simulink library "xps_library"  (R2018a)
settings: Solver=ode45  StartTime=0.0  StopTime=10.0  RelTol=1e-3
undefined symbols (not defined in the file or in its folder): ip_name, lib_path
libraries: xbsIndex_r4 x2454, casper_library_flow_control x68, simulink x52, $bdroot x22, casper_library_misc x9
(part 3 of 27)

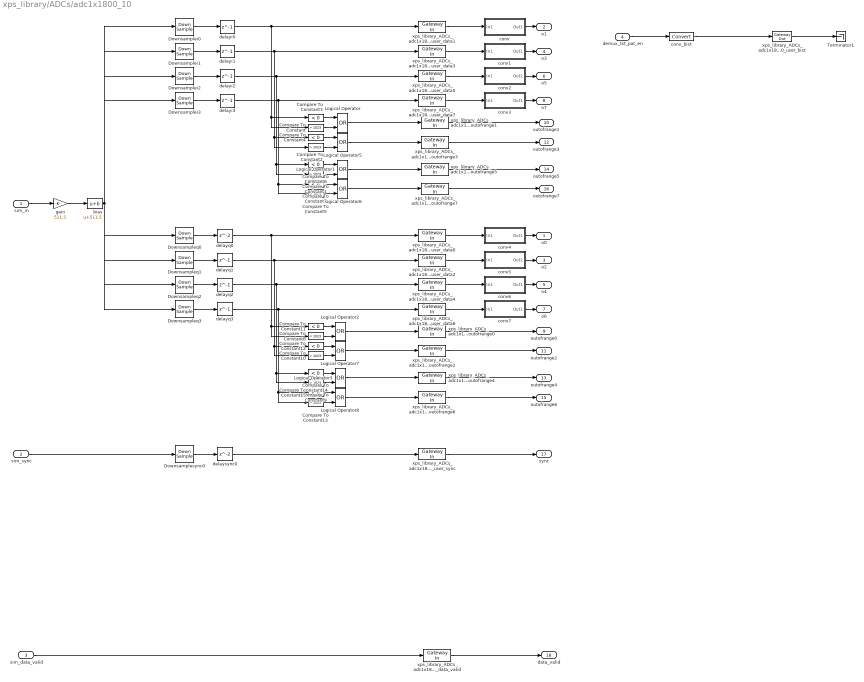
== system xps_library/ADCs/adc1x1800_10 ==
  sim_in : Inport  SampleTime=sample_period/8
  sim_sync : Inport  Port=2  SampleTime=sample_period/8
  sim_data_valid : Inport  Port=3  SampleTime=sample_period/4
  demux_tst_pat_en : Inport  Port=4  SampleTime=sample_period/8
  Compare To Constant{,1..2,5,8..10,13} (8 alike) : simulink/Logic and Bit Operations/Compare To Constant  relop=>  const=1023  OutDataTypeStr=boolean  ZeroCross=off
  Compare To Constant{3..4,6..7,11..12,14..15} (8 alike) : simulink/Logic and Bit Operations/Compare To Constant  relop=<  const=0  OutDataTypeStr=boolean  ZeroCross=off
  Downsamplei0 : DownSample  N=8  phase=1  InputProcessing=Inherited (this choice will be removed - see release notes)
  Downsamplei1 : DownSample  N=8  phase=3  InputProcessing=Inherited (this choice will be removed - see release notes)
  Downsamplei2 : DownSample  N=8  phase=5  InputProcessing=Inherited (this choice will be removed - see release notes)
  Downsamplei3 : DownSample  N=8  phase=7  InputProcessing=Inherited (this choice will be removed - see release notes)
  Downsampleq0 : DownSample  N=8  InputProcessing=Inherited (this choice will be removed - see release notes)
  Downsampleq1 : DownSample  N=8  phase=2  InputProcessing=Inherited (this choice will be removed - see release notes)
  Downsampleq2 : DownSample  N=8  phase=4  InputProcessing=Inherited (this choice will be removed - see release notes)
  Downsampleq3 : DownSample  N=8  phase=6  InputProcessing=Inherited (this choice will be removed - see release notes)
  Downsamplesync0 : DownSample  N=8  InputProcessing=Inherited (this choice will be removed - see release notes)
  Logical Operator{,1..3,5..8} (8 alike) : Logic  Operator=OR  AllPortsSameDT=off  OutDataTypeStr=boolean
  Terminator1 : Terminator
  bias : Bias  Bias=511.5  SaturateOnIntegerOverflow=on
  conv : Subsystem
  conv1 : Subsystem
  conv2 : Subsystem
  conv3 : Subsystem
  conv4 : Subsystem
  conv5 : Subsystem
  conv6 : Subsystem
  conv7 : Subsystem
  conv_bist : xbsIndex_r4/Convert  gui_display_data_type=Fixed-point  arith_type=Boolean  n_bits=8  bin_pt=0  float_type=Single  exp_bits=8  fraction_bits=24  quantization=Truncate  overflow=Wrap  en=off  latency=0  pipeline=off  dbl_ovrd=off  block_type=convert
      settings: xl_area=[0, 0, 0, 0, 0, 0, 0]
  delayi{0..3} (4 alike) : Delay  DelayLength=1  InputProcessing=Inherited
  delayq0 : Delay  InputProcessing=Inherited
  delayq1 : Delay  DelayLength=1  InputProcessing=Inherited
  delayq2 : Delay  DelayLength=1  InputProcessing=Inherited
  delayq3 : Delay  DelayLength=1  InputProcessing=Inherited
  delaysync0 : Delay  InputProcessing=Inherited
  gain : Gain  Gain=511.5  SaturateOnIntegerOverflow=on  OutDataTypeStr=Inherit: Same as input  ParamDataTypeStr=Inherit: Same as input
  xps_library_ADCs_adc1x1800_10_user_bist : xbsIndex_r4/Gateway Out  inherit_from_input=off  hdl_port=on  rows=1  columns=1  UseAsDAC=off  DACChannel='1'  interface=None  automatic_assignment=on  address_offset=hex2dec('00')  intf_name=''  intf_description=''  timing_constraint=None  locs_specified=off  LOCs={}  io_standard={}  block_type=gatewayout
      settings: infoedit="Gateway out block.  Converts Xilinx fixed point inputs into ouputs of type Simulink integer, double, or fixed point.<br><br>Hardware notes:  In hardware these blocks become top level output ports or are discarded, depending on how they are configured."  block_version=11.4
  xps_library_ADCs_adc1x1800_10_user_data{0..7} (8 alike) : xbsIndex_r4/Gateway In  gui_display_data_type=Fixed-point  arith_type=Unsigned  n_bits=10  bin_pt=0  preci_type=Single  exp_width=8  frac_width=24  rows=1  columns=1  quantization="Round  (unbiased: +/- Inf)"  overflow=Saturate  period=sample_period  UseAsADC=off  ADCChannel='1'  interface=None  automatic_assignment=on  address_offset=hex2dec('00')  intf_name=''  intf_description=''  default_value=0  timing_constraint=None  locs_specified=off  LOCs={}  io_standard={}  inherit_from_input=off  hdl_port=on  dbl_ovrd=off  block_type=gatewayin
      settings: infoedit="Gateway in block.  Converts inputs of type Simulink integer, double and fixed point to  Xilinx fixed point type.<br><br>Hardware notes:  In hardware these blocks become top level input ports."  xl_area=[0 0 0 0 8 0 0]  block_version=8.2.02
  xps_library_ADCs_adc1x1800_10_user_data_valid : xbsIndex_r4/Gateway In  gui_display_data_type=Fixed-point  arith_type=Boolean  n_bits=8  bin_pt=0  preci_type=Single  exp_width=8  frac_width=24  rows=1  columns=1  quantization="Round  (unbiased: +/- Inf)"  overflow=Saturate  period=sample_period  UseAsADC=off  ADCChannel='1'  interface=None  automatic_assignment=on  address_offset=hex2dec('00')  intf_name=''  intf_description=''  default_value=0  timing_constraint=None  locs_specified=off  LOCs={}  io_standard={}  inherit_from_input=off  hdl_port=on  dbl_ovrd=off  block_type=gatewayin
      settings: infoedit="Gateway in block.  Converts inputs of type Simulink integer, double and fixed point to  Xilinx fixed point type.<P><P>Hardware notes:  In hardware these blocks become top level input ports."  xl_area=[0 0 0 0 8 0 0]  block_version=8.2.02
  xps_library_ADCs_adc1x1800_10_user_outofrange{0..7} (8 alike) : xbsIndex_r4/Gateway In  gui_display_data_type=Fixed-point  arith_type=Boolean  n_bits=8  bin_pt=0  preci_type=Single  exp_width=8  frac_width=24  rows=1  columns=1  quantization="Round  (unbiased: +/- Inf)"  overflow=Saturate  period=sample_period  UseAsADC=off  ADCChannel='1'  interface=None  automatic_assignment=on  address_offset=hex2dec('00')  intf_name=''  intf_description=''  default_value=0  timing_constraint=None  locs_specified=off  LOCs={}  io_standard={}  inherit_from_input=off  hdl_port=on  dbl_ovrd=off  block_type=gatewayin
      settings: infoedit="Gateway in block.  Converts inputs of type Simulink integer, double and fixed point to  Xilinx fixed point type.<P><P>Hardware notes:  In hardware these blocks become top level input ports."  xl_area=[0 0 0 0 8 0 0]  block_version=8.2.02
  xps_library_ADCs_adc1x1800_10_user_sync : xbsIndex_r4/Gateway In  gui_display_data_type=Fixed-point  arith_type=Boolean  n_bits=8  bin_pt=0  preci_type=Single  exp_width=8  frac_width=24  rows=1  columns=1  quantization="Round  (unbiased: +/- Inf)"  overflow=Saturate  period=sample_period  UseAsADC=off  ADCChannel='1'  interface=None  automatic_assignment=on  address_offset=hex2dec('00')  intf_name=''  intf_description=''  default_value=0  timing_constraint=None  locs_specified=off  LOCs={}  io_standard={}  inherit_from_input=off  hdl_port=on  dbl_ovrd=off  block_type=gatewayin
      settings: infoedit="Gateway in block.  Converts inputs of type Simulink integer, double and fixed point to  Xilinx fixed point type.<P><P>Hardware notes:  In hardware these blocks become top level input ports."  xl_area=[0 0 0 0 8 0 0]  block_version=8.2.02
  o0 : Outport
  o1 : Outport  Port=2
  o2 : Outport  Port=3
  o3 : Outport  Port=4
  o4 : Outport  Port=5
  o5 : Outport  Port=6
  o6 : Outport  Port=7
  o7 : Outport  Port=8
  outofrange0 : Outport  Port=9
  outofrange1 : Outport  Port=10
  outofrange2 : Outport  Port=11
  outofrange3 : Outport  Port=12
  outofrange4 : Outport  Port=13
  outofrange5 : Outport  Port=14
  outofrange6 : Outport  Port=15
  outofrange7 : Outport  Port=16
  sync : Outport  Port=17
  data_valid : Outport  Port=18
  wires:
  delayq3/1 -> xps_library_ADCs_adc1x1800_10_user_data6/1, Compare To Constant15/1, Compare To Constant13/1
  delayq2/1 -> xps_library_ADCs_adc1x1800_10_user_data4/1, Compare To Constant14/1, Compare To Constant9/1
  delayq1/1 -> xps_library_ADCs_adc1x1800_10_user_data2/1, Compare To Constant12/1, Compare To Constant10/1
  delayi3/1 -> xps_library_ADCs_adc1x1800_10_user_data7/1, Compare To Constant7/1, Compare To Constant5/1
  delayi2/1 -> xps_library_ADCs_adc1x1800_10_user_data5/1, Compare To Constant6/1, Compare To Constant1/1
  delayi1/1 -> xps_library_ADCs_adc1x1800_10_user_data3/1, Compare To Constant2/1, Compare To Constant4/1
  Downsamplei0/1 -> delayi0/1
  xps_library_ADCs_adc1x1800_10_user_data6/1 -> conv7/1(In1)
  xps_library_ADCs_adc1x1800_10_user_data4/1 -> conv6/1(In1)
  xps_library_ADCs_adc1x1800_10_user_data2/1 -> conv5/1(In1)
  xps_library_ADCs_adc1x1800_10_user_data0/1 -> conv4/1(In1)
  xps_library_ADCs_adc1x1800_10_user_sync/1 -> sync/1
  xps_library_ADCs_adc1x1800_10_user_outofrange1/1 -> outofrange1/1
  xps_library_ADCs_adc1x1800_10_user_data7/1 -> conv3/1(In1)
  xps_library_ADCs_adc1x1800_10_user_data5/1 -> conv2/1(In1)
  xps_library_ADCs_adc1x1800_10_user_data3/1 -> conv1/1(In1)
  Downsampleq3/1 -> delayq3/1
  Downsampleq2/1 -> delayq2/1
  Downsampleq1/1 -> delayq1/1
  Downsamplei3/1 -> delayi3/1
  Downsamplei2/1 -> delayi2/1
  Downsamplei1/1 -> delayi1/1
  delayi0/1 -> xps_library_ADCs_adc1x1800_10_user_data1/1, Compare To Constant/1, Compare To Constant3/1
  Downsampleq0/1 -> delayq0/1
  delayq0/1 -> xps_library_ADCs_adc1x1800_10_user_data0/1, Compare To Constant11/1, Compare To Constant8/1
  Compare To Constant3/1 -> Logical Operator/1
  Compare To Constant/1 -> Logical Operator/2
  Compare To Constant4/1 -> Logical Operator5/1
  Compare To Constant2/1 -> Logical Operator5/2
  Logical Operator/1 -> xps_library_ADCs_adc1x1800_10_user_outofrange1/1
  Compare To Constant6/1 -> Logical Operator1/1
  Compare To Constant1/1 -> Logical Operator1/2
  Compare To Constant7/1 -> Logical Operator6/1
  Compare To Constant5/1 -> Logical Operator6/2
  Compare To Constant11/1 -> Logical Operator2/1
  Compare To Constant8/1 -> Logical Operator2/2
  Compare To Constant12/1 -> Logical Operator7/1
  Compare To Constant10/1 -> Logical Operator7/2
  Compare To Constant14/1 -> Logical Operator3/1
  Compare To Constant9/1 -> Logical Operator3/2
  Compare To Constant15/1 -> Logical Operator8/1
  Compare To Constant13/1 -> Logical Operator8/2
  sim_sync/1 -> Downsamplesync0/1
  Downsamplesync0/1 -> delaysync0/1
  delaysync0/1 -> xps_library_ADCs_adc1x1800_10_user_sync/1
  xps_library_ADCs_adc1x1800_10_user_data1/1 -> conv/1(In1)
  sim_in/1 -> gain/1
  gain/1 -> bias/1
  bias/1 -> Downsamplei0/1, Downsamplei1/1, Downsamplei2/1, Downsamplei3/1, Downsampleq0/1, Downsampleq1/1, Downsampleq2/1, Downsampleq3/1
  xps_library_ADCs_adc1x1800_10_user_outofrange3/1 -> outofrange3/1
  Logical Operator5/1 -> xps_library_ADCs_adc1x1800_10_user_outofrange3/1
  xps_library_ADCs_adc1x1800_10_user_outofrange5/1 -> outofrange5/1
  Logical Operator1/1 -> xps_library_ADCs_adc1x1800_10_user_outofrange5/1
  xps_library_ADCs_adc1x1800_10_user_outofrange7/1 -> outofrange7/1
  Logical Operator6/1 -> xps_library_ADCs_adc1x1800_10_user_outofrange7/1
  xps_library_ADCs_adc1x1800_10_user_outofrange0/1 -> outofrange0/1
  Logical Operator2/1 -> xps_library_ADCs_adc1x1800_10_user_outofrange0/1
  xps_library_ADCs_adc1x1800_10_user_outofrange2/1 -> outofrange2/1
  Logical Operator7/1 -> xps_library_ADCs_adc1x1800_10_user_outofrange2/1
  xps_library_ADCs_adc1x1800_10_user_outofrange4/1 -> outofrange4/1
  Logical Operator3/1 -> xps_library_ADCs_adc1x1800_10_user_outofrange4/1
  xps_library_ADCs_adc1x1800_10_user_outofrange6/1 -> outofrange6/1
  Logical Operator8/1 -> xps_library_ADCs_adc1x1800_10_user_outofrange6/1
  xps_library_ADCs_adc1x1800_10_user_data_valid/1 -> data_valid/1
  sim_data_valid/1 -> xps_library_ADCs_adc1x1800_10_user_data_valid/1
  demux_tst_pat_en/1 -> conv_bist/1
  xps_library_ADCs_adc1x1800_10_user_bist/1 -> Terminator1/1
  conv_bist/1 -> xps_library_ADCs_adc1x1800_10_user_bist/1
  conv/1(Out1) -> o1/1
  conv1/1(Out1) -> o3/1
  conv2/1(Out1) -> o5/1
  conv3/1(Out1) -> o7/1
  conv4/1(Out1) -> o0/1
  conv5/1(Out1) -> o2/1
  conv6/1(Out1) -> o4/1
  conv7/1(Out1) -> o6/1

== system xps_library/ADCs/adc2x14_400 ==
  conv : Subsystem
      mask help:
      | Converts an (12-bit) unsigned number to 2's complement.
      | This block should eventually be able to handle arbitrary
      | width inputs.
  conv1 : Subsystem
      mask help:
      | Converts an (12-bit) unsigned number to 2's complement.
      | This block should eventually be able to handle arbitrary
      | width inputs.
  conv2 : Subsystem
      mask help:
      | Converts an (12-bit) unsigned number to 2's complement.
      | This block should eventually be able to handle arbitrary
      | width inputs.
  conv3 : Subsystem
      mask help:
      | Converts an (12-bit) unsigned number to 2's complement.
      | This block should eventually be able to handle arbitrary
      | width inputs.
  xps_library_ADCs_adc2x14_400_user_data_i0 : xbsIndex_r4/Gateway In  gui_display_data_type=Fixed-point  arith_type=Unsigned  n_bits=14  bin_pt=0  preci_type=Single  exp_width=8  frac_width=24  rows=1  columns=1  quantization=Truncate  overflow=Wrap  period=1  UseAsADC=off  ADCChannel='1'  interface=None  automatic_assignment=on  address_offset=hex2dec('00')  intf_name=''  intf_description=''  default_value=0  timing_constraint=None  locs_specified=off  LOCs={}  io_standard={}  inherit_from_input=off  hdl_port=on  dbl_ovrd=off  block_type=gatewayin
      settings: infoedit="Gateway in block.  Converts inputs of type Simulink integer, double and fixed point to  Xilinx fixed point type.<P><P>Hardware notes:  In hardware these blocks become top level input ports."  xl_area=[0, 0, 0, 0, 0, 0, 0]  block_version=10.1.3
  xps_library_ADCs_adc2x14_400_user_data_i1 : xbsIndex_r4/Gateway In  gui_display_data_type=Fixed-point  arith_type=Unsigned  n_bits=14  bin_pt=0  preci_type=Single  exp_width=8  frac_width=24  rows=1  columns=1  quantization=Truncate  overflow=Wrap  period=1  UseAsADC=off  ADCChannel='1'  interface=None  automatic_assignment=on  address_offset=hex2dec('00')  intf_name=''  intf_description=''  default_value=0  timing_constraint=None  locs_specified=off  LOCs={}  io_standard={}  inherit_from_input=off  hdl_port=on  dbl_ovrd=off  block_type=gatewayin
      settings: infoedit="Gateway in block.  Converts inputs of type Simulink integer, double and fixed point to  Xilinx fixed point type.<P><P>Hardware notes:  In hardware these blocks become top level input ports."  xl_area=[0, 0, 0, 0, 0, 0, 0]  block_version=10.1.3
  xps_library_ADCs_adc2x14_400_user_data_q0 : xbsIndex_r4/Gateway In  gui_display_data_type=Fixed-point  arith_type=Unsigned  n_bits=14  bin_pt=0  preci_type=Single  exp_width=8  frac_width=24  rows=1  columns=1  quantization=Truncate  overflow=Wrap  period=1  UseAsADC=off  ADCChannel='1'  interface=None  automatic_assignment=on  address_offset=hex2dec('00')  intf_name=''  intf_description=''  default_value=0  timing_constraint=None  locs_specified=off  LOCs={}  io_standard={}  inherit_from_input=off  hdl_port=on  dbl_ovrd=off  block_type=gatewayin
      settings: infoedit="Gateway in block.  Converts inputs of type Simulink integer, double and fixed point to  Xilinx fixed point type.<P><P>Hardware notes:  In hardware these blocks become top level input ports."  xl_area=[0, 0, 0, 0, 0, 0, 0]  block_version=10.1.3
  xps_library_ADCs_adc2x14_400_user_data_q1 : xbsIndex_r4/Gateway In  gui_display_data_type=Fixed-point  arith_type=Unsigned  n_bits=14  bin_pt=0  preci_type=Single  exp_width=8  frac_width=24  rows=1  columns=1  quantization=Truncate  overflow=Wrap  period=1  UseAsADC=off  ADCChannel='1'  interface=None  automatic_assignment=on  address_offset=hex2dec('00')  intf_name=''  intf_description=''  default_value=0  timing_constraint=None  locs_specified=off  LOCs={}  io_standard={}  inherit_from_input=off  hdl_port=on  dbl_ovrd=off  block_type=gatewayin
      settings: infoedit="Gateway in block.  Converts inputs of type Simulink integer, double and fixed point to  Xilinx fixed point type.<P><P>Hardware notes:  In hardware these blocks become top level input ports."  xl_area=[0, 0, 0, 0, 0, 0, 0]  block_version=10.1.3
  xps_library_ADCs_adc2x14_400_user_sync : xbsIndex_r4/Gateway In  gui_display_data_type=Fixed-point  arith_type=Boolean  n_bits=1  bin_pt=0  preci_type=Single  exp_width=8  frac_width=24  rows=1  columns=1  quantization=Truncate  overflow=Wrap  period=1  UseAsADC=off  ADCChannel='1'  interface=None  automatic_assignment=on  address_offset=hex2dec('00')  intf_name=''  intf_description=''  default_value=0  timing_constraint=None  locs_specified=off  LOCs={}  io_standard={}  inherit_from_input=off  hdl_port=on  dbl_ovrd=off  block_type=gatewayin
      settings: infoedit="Gateway in block.  Converts inputs of type Simulink integer, double and fixed point to  Xilinx fixed point type.<P><P>Hardware notes:  In hardware these blocks become top level input ports."  xl_area=[0, 0, 0, 0, 0, 0, 0]  block_version=10.1.3
  data_i0 : Outport
  data_i1 : Outport  Port=2
  data_q0 : Outport  Port=3
  data_q1 : Outport  Port=4
  sync : Outport  Port=5
  wires:
  xps_library_ADCs_adc2x14_400_user_sync/1 -> sync/1
  xps_library_ADCs_adc2x14_400_user_data_i0/1 -> conv/1(In1)
  conv/1(Out1) -> data_i0/1
  xps_library_ADCs_adc2x14_400_user_data_q0/1 -> conv2/1(In1)
  conv2/1(Out1) -> data_q0/1
  xps_library_ADCs_adc2x14_400_user_data_i1/1 -> conv1/1(In1)
  conv1/1(Out1) -> data_i1/1
  xps_library_ADCs_adc2x14_400_user_data_q1/1 -> conv3/1(In1)
  conv3/1(Out1) -> data_q1/1

== system xps_library/ADCs/adc2x14_400_4x ==
  conv : Subsystem
      mask help:
      | Converts an (14-bit) unsigned number to 2's complement.
      | This block should eventually be able to handle arbitrary
      | width inputs.
  conv1 : Subsystem
      mask help:
      | Converts an (14-bit) unsigned number to 2's complement.
      | This block should eventually be able to handle arbitrary
      | width inputs.
  conv2 : Subsystem
      mask help:
      | Converts an (14-bit) unsigned number to 2's complement.
      | This block should eventually be able to handle arbitrary
      | width inputs.
  conv3 : Subsystem
      mask help:
      | Converts an (14-bit) unsigned number to 2's complement.
      | This block should eventually be able to handle arbitrary
      | width inputs.
  conv4 : Subsystem
      mask help:
      | Converts an (14-bit) unsigned number to 2's complement.
      | This block should eventually be able to handle arbitrary
      | width inputs.
  conv5 : Subsystem
      mask help:
      | Converts an (14-bit) unsigned number to 2's complement.
      | This block should eventually be able to handle arbitrary
      | width inputs.
  conv6 : Subsystem
      mask help:
      | Converts an (14-bit) unsigned number to 2's complement.
      | This block should eventually be able to handle arbitrary
      | width inputs.
  conv7 : Subsystem
      mask help:
      | Converts an (14-bit) unsigned number to 2's complement.
      | This block should eventually be able to handle arbitrary
      | width inputs.
  xps_library_ADCs_adc2x14_400_4x_user_data_i{0..3} (4 alike) : xbsIndex_r4/Gateway In  gui_display_data_type=Fixed-point  arith_type=Unsigned  n_bits=14  bin_pt=0  preci_type=Single  exp_width=8  frac_width=24  rows=1  columns=1  quantization=Truncate  overflow=Wrap  period=1  UseAsADC=off  ADCChannel='1'  interface=None  automatic_assignment=on  address_offset=hex2dec('00')  intf_name=''  intf_description=''  default_value=0  timing_constraint=None  locs_specified=off  LOCs={}  io_standard={}  inherit_from_input=off  hdl_port=on  dbl_ovrd=off  block_type=gatewayin
      settings: infoedit="Gateway in block.  Converts inputs of type Simulink integer, double and fixed point to  Xilinx fixed point type.<P><P>Hardware notes:  In hardware these blocks become top level input ports."  xl_area=[0, 0, 0, 0, 0, 0, 0]  block_version=10.1.3
  xps_library_ADCs_adc2x14_400_4x_user_data_q{0..3} (4 alike) : xbsIndex_r4/Gateway In  gui_display_data_type=Fixed-point  arith_type=Unsigned  n_bits=14  bin_pt=0  preci_type=Single  exp_width=8  frac_width=24  rows=1  columns=1  quantization=Truncate  overflow=Wrap  period=1  UseAsADC=off  ADCChannel='1'  interface=None  automatic_assignment=on  address_offset=hex2dec('00')  intf_name=''  intf_description=''  default_value=0  timing_constraint=None  locs_specified=off  LOCs={}  io_standard={}  inherit_from_input=off  hdl_port=on  dbl_ovrd=off  block_type=gatewayin
      settings: infoedit="Gateway in block.  Converts inputs of type Simulink integer, double and fixed point to  Xilinx fixed point type.<P><P>Hardware notes:  In hardware these blocks become top level input ports."  xl_area=[0, 0, 0, 0, 0, 0, 0]  block_version=10.1.3
  xps_library_ADCs_adc2x14_400_4x_user_sync : xbsIndex_r4/Gateway In  gui_display_data_type=Fixed-point  arith_type=Boolean  n_bits=1  bin_pt=0  preci_type=Single  exp_width=8  frac_width=24  rows=1  columns=1  quantization=Truncate  overflow=Wrap  period=1  UseAsADC=off  ADCChannel='1'  interface=None  automatic_assignment=on  address_offset=hex2dec('00')  intf_name=''  intf_description=''  default_value=0  timing_constraint=None  locs_specified=off  LOCs={}  io_standard={}  inherit_from_input=off  hdl_port=on  dbl_ovrd=off  block_type=gatewayin
      settings: infoedit="Gateway in block.  Converts inputs of type Simulink integer, double and fixed point to  Xilinx fixed point type.<P><P>Hardware notes:  In hardware these blocks become top level input ports."  xl_area=[0, 0, 0, 0, 0, 0, 0]  block_version=10.1.3
  data_i0 : Outport
  data_i1 : Outport  Port=2
  data_i2 : Outport  Port=3
  data_i3 : Outport  Port=4
  data_q0 : Outport  Port=5
  data_q1 : Outport  Port=6
  data_q2 : Outport  Port=7
  data_q3 : Outport  Port=8
  sync : Outport  Port=9
  wires:
  conv5/1(Out1) -> data_q1/1
  xps_library_ADCs_adc2x14_400_4x_user_data_q1/1 -> conv5/1(In1)
  conv1/1(Out1) -> data_i1/1
  xps_library_ADCs_adc2x14_400_4x_user_data_i1/1 -> conv1/1(In1)
  conv4/1(Out1) -> data_q0/1
  xps_library_ADCs_adc2x14_400_4x_user_data_q0/1 -> conv4/1(In1)
  conv/1(Out1) -> data_i0/1
  xps_library_ADCs_adc2x14_400_4x_user_data_i0/1 -> conv/1(In1)
  xps_library_ADCs_adc2x14_400_4x_user_sync/1 -> sync/1
  conv2/1(Out1) -> data_i2/1
  xps_library_ADCs_adc2x14_400_4x_user_data_i2/1 -> conv2/1(In1)
  conv3/1(Out1) -> data_i3/1
  xps_library_ADCs_adc2x14_400_4x_user_data_i3/1 -> conv3/1(In1)
  conv6/1(Out1) -> data_q2/1
  xps_library_ADCs_adc2x14_400_4x_user_data_q2/1 -> conv6/1(In1)
  conv7/1(Out1) -> data_q3/1
  xps_library_ADCs_adc2x14_400_4x_user_data_q3/1 -> conv7/1(In1)

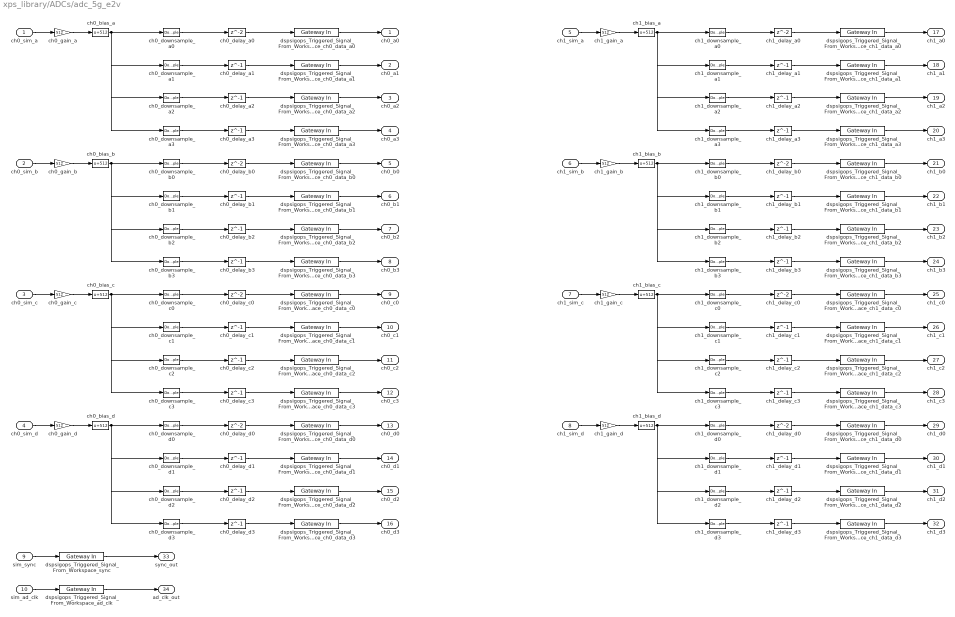
== system xps_library/ADCs/adc_5g_e2v ==
  ch0_sim_a : Inport
  ch0_sim_b : Inport  Port=2
  ch0_sim_c : Inport  Port=3
  ch0_sim_d : Inport  Port=4
  ch1_sim_a : Inport  Port=5
  ch1_sim_b : Inport  Port=6
  ch1_sim_c : Inport  Port=7
  ch1_sim_d : Inport  Port=8
  sim_sync : Inport  Port=9
  sim_ad_clk : Inport  Port=10
  ch0_bias_a : Bias  Bias=512  SaturateOnIntegerOverflow=on
  ch0_bias_b : Bias  Bias=512  SaturateOnIntegerOverflow=on
  ch0_bias_c : Bias  Bias=512  SaturateOnIntegerOverflow=on
  ch0_bias_d : Bias  Bias=512  SaturateOnIntegerOverflow=on
  ch0_delay_a0 : Delay  InitialCondition=0  InputProcessing=Inherited
  ch0_delay_a1 : Delay  DelayLength=1  InitialCondition=0  InputProcessing=Inherited
  ch0_delay_a2 : Delay  DelayLength=1  InitialCondition=0  InputProcessing=Inherited
  ch0_delay_a3 : Delay  DelayLength=1  InitialCondition=0  InputProcessing=Inherited
  ch0_delay_b0 : Delay  InitialCondition=0  InputProcessing=Inherited
  ch0_delay_b1 : Delay  DelayLength=1  InitialCondition=0  InputProcessing=Inherited
  ch0_delay_b2 : Delay  DelayLength=1  InitialCondition=0  InputProcessing=Inherited
  ch0_delay_b3 : Delay  DelayLength=1  InitialCondition=0  InputProcessing=Inherited
  ch0_delay_c0 : Delay  InitialCondition=0  InputProcessing=Inherited
  ch0_delay_c1 : Delay  DelayLength=1  InitialCondition=0  InputProcessing=Inherited
  ch0_delay_c2 : Delay  DelayLength=1  InitialCondition=0  InputProcessing=Inherited
  ch0_delay_c3 : Delay  DelayLength=1  InitialCondition=0  InputProcessing=Inherited
  ch0_delay_d0 : Delay  InitialCondition=0  InputProcessing=Inherited
  ch0_delay_d1 : Delay  DelayLength=1  InitialCondition=0  InputProcessing=Inherited
  ch0_delay_d2 : Delay  DelayLength=1  InitialCondition=0  InputProcessing=Inherited
  ch0_delay_d3 : Delay  DelayLength=1  InitialCondition=0  InputProcessing=Inherited
  ch0_downsample_a0 : DownSample  N=4  RateOptions=Allow multirate processing
  ch0_downsample_a1 : DownSample  N=4  phase=1  RateOptions=Allow multirate processing
  ch0_downsample_a2 : DownSample  N=4  phase=2  RateOptions=Allow multirate processing
  ch0_downsample_a3 : DownSample  N=4  phase=3  RateOptions=Allow multirate processing
  ch0_downsample_b0 : DownSample  N=4  RateOptions=Allow multirate processing
  ch0_downsample_b1 : DownSample  N=4  phase=1  RateOptions=Allow multirate processing
  ch0_downsample_b2 : DownSample  N=4  phase=2  RateOptions=Allow multirate processing
  ch0_downsample_b3 : DownSample  N=4  phase=3  RateOptions=Allow multirate processing
  ch0_downsample_c0 : DownSample  N=4  RateOptions=Allow multirate processing
  ch0_downsample_c1 : DownSample  N=4  phase=1  RateOptions=Allow multirate processing
  ch0_downsample_c2 : DownSample  N=4  phase=2  RateOptions=Allow multirate processing
  ch0_downsample_c3 : DownSample  N=4  phase=3  RateOptions=Allow multirate processing
  ch0_downsample_d0 : DownSample  N=4  RateOptions=Allow multirate processing
  ch0_downsample_d1 : DownSample  N=4  phase=1  RateOptions=Allow multirate processing
  ch0_downsample_d2 : DownSample  N=4  phase=2  RateOptions=Allow multirate processing
  ch0_downsample_d3 : DownSample  N=4  phase=3  RateOptions=Allow multirate processing
  ch0_gain_a : Gain  Gain=512  SaturateOnIntegerOverflow=on  OutDataTypeStr=Inherit: Same as input  ParamDataTypeStr=Inherit: Same as input
  ch0_gain_b : Gain  Gain=512  SaturateOnIntegerOverflow=on  OutDataTypeStr=Inherit: Same as input  ParamDataTypeStr=Inherit: Same as input
  ch0_gain_c : Gain  Gain=512  SaturateOnIntegerOverflow=on  OutDataTypeStr=Inherit: Same as input  ParamDataTypeStr=Inherit: Same as input
  ch0_gain_d : Gain  Gain=512  SaturateOnIntegerOverflow=on  OutDataTypeStr=Inherit: Same as input  ParamDataTypeStr=Inherit: Same as input
  ch1_bias_a : Bias  Bias=512  SaturateOnIntegerOverflow=on
  ch1_bias_b : Bias  Bias=512  SaturateOnIntegerOverflow=on
  ch1_bias_c : Bias  Bias=512  SaturateOnIntegerOverflow=on
  ch1_bias_d : Bias  Bias=512  SaturateOnIntegerOverflow=on
  ch1_delay_a0 : Delay  InitialCondition=0  InputProcessing=Inherited
  ch1_delay_a1 : Delay  DelayLength=1  InitialCondition=0  InputProcessing=Inherited
  ch1_delay_a2 : Delay  DelayLength=1  InitialCondition=0  InputProcessing=Inherited
  ch1_delay_a3 : Delay  DelayLength=1  InitialCondition=0  InputProcessing=Inherited
  ch1_delay_b0 : Delay  InitialCondition=0  InputProcessing=Inherited
  ch1_delay_b1 : Delay  DelayLength=1  InitialCondition=0  InputProcessing=Inherited
  ch1_delay_b2 : Delay  DelayLength=1  InitialCondition=0  InputProcessing=Inherited
  ch1_delay_b3 : Delay  DelayLength=1  InitialCondition=0  InputProcessing=Inherited
  ch1_delay_c0 : Delay  InitialCondition=0  InputProcessing=Inherited
  ch1_delay_c1 : Delay  DelayLength=1  InitialCondition=0  InputProcessing=Inherited
  ch1_delay_c2 : Delay  DelayLength=1  InitialCondition=0  InputProcessing=Inherited
  ch1_delay_c3 : Delay  DelayLength=1  InitialCondition=0  InputProcessing=Inherited
  ch1_delay_d0 : Delay  InitialCondition=0  InputProcessing=Inherited
  ch1_delay_d1 : Delay  DelayLength=1  InitialCondition=0  InputProcessing=Inherited
  ch1_delay_d2 : Delay  DelayLength=1  InitialCondition=0  InputProcessing=Inherited
  ch1_delay_d3 : Delay  DelayLength=1  InitialCondition=0  InputProcessing=Inherited
  ch1_downsample_a0 : DownSample  N=4  RateOptions=Allow multirate processing
  ch1_downsample_a1 : DownSample  N=4  phase=1  RateOptions=Allow multirate processing
  ch1_downsample_a2 : DownSample  N=4  phase=2  RateOptions=Allow multirate processing
  ch1_downsample_a3 : DownSample  N=4  phase=3  RateOptions=Allow multirate processing
  ch1_downsample_b0 : DownSample  N=4  RateOptions=Allow multirate processing
  ch1_downsample_b1 : DownSample  N=4  phase=1  RateOptions=Allow multirate processing
  ch1_downsample_b2 : DownSample  N=4  phase=2  RateOptions=Allow multirate processing
  ch1_downsample_b3 : DownSample  N=4  phase=3  RateOptions=Allow multirate processing
  ch1_downsample_c0 : DownSample  N=4  RateOptions=Allow multirate processing
  ch1_downsample_c1 : DownSample  N=4  phase=1  RateOptions=Allow multirate processing
  ch1_downsample_c2 : DownSample  N=4  phase=2  RateOptions=Allow multirate processing
  ch1_downsample_c3 : DownSample  N=4  phase=3  RateOptions=Allow multirate processing
  ch1_downsample_d0 : DownSample  N=4  RateOptions=Allow multirate processing
  ch1_downsample_d1 : DownSample  N=4  phase=1  RateOptions=Allow multirate processing
  ch1_downsample_d2 : DownSample  N=4  phase=2  RateOptions=Allow multirate processing
  ch1_downsample_d3 : DownSample  N=4  phase=3  RateOptions=Allow multirate processing
  ch1_gain_a : Gain  Gain=512  SaturateOnIntegerOverflow=on  OutDataTypeStr=Inherit: Same as input  ParamDataTypeStr=Inherit: Same as input
  ch1_gain_b : Gain  Gain=512  SaturateOnIntegerOverflow=on  OutDataTypeStr=Inherit: Same as input  ParamDataTypeStr=Inherit: Same as input
  ch1_gain_c : Gain  Gain=512  SaturateOnIntegerOverflow=on  OutDataTypeStr=Inherit: Same as input  ParamDataTypeStr=Inherit: Same as input
  ch1_gain_d : Gain  Gain=512  SaturateOnIntegerOverflow=on  OutDataTypeStr=Inherit: Same as input  ParamDataTypeStr=Inherit: Same as input
  dspsigops_Triggered_Signal_From_Workspace_ad_clk : xbsIndex_r4/Gateway In  gui_display_data_type=Fixed-point  arith_type=Boolean  n_bits=16  bin_pt=14  preci_type=Single  exp_width=8  frac_width=24  rows=1  columns=1  quantization="Round  (unbiased: +/- Inf)"  overflow=Saturate  period=1  UseAsADC=off  ADCChannel='1'  interface=None  automatic_assignment=on  address_offset=hex2dec('00')  intf_name=''  intf_description=''  default_value=0  timing_constraint=None  locs_specified=off  LOCs={}  io_standard={}  inherit_from_input=off  hdl_port=on  dbl_ovrd=off  block_type=gatewayin
  dspsigops_Triggered_Signal_From_Workspace_ch0_data_a{0..3} (4 alike) : xbsIndex_r4/Gateway In  gui_display_data_type=Fixed-point  arith_type=Unsigned  n_bits=10  bin_pt=0  preci_type=Single  exp_width=8  frac_width=24  rows=1  columns=1  quantization=Truncate  overflow=Wrap  period=1  UseAsADC=off  ADCChannel='1'  interface=None  automatic_assignment=on  address_offset=hex2dec('00')  intf_name=''  intf_description=''  default_value=0  timing_constraint=None  locs_specified=off  LOCs={}  io_standard={}  inherit_from_input=off  hdl_port=on  dbl_ovrd=off  block_type=gatewayin
  dspsigops_Triggered_Signal_From_Workspace_ch0_data_b{0..3} (4 alike) : xbsIndex_r4/Gateway In  gui_display_data_type=Fixed-point  arith_type=Unsigned  n_bits=10  bin_pt=0  preci_type=Single  exp_width=8  frac_width=24  rows=1  columns=1  quantization=Truncate  overflow=Wrap  period=1  UseAsADC=off  ADCChannel='1'  interface=None  automatic_assignment=on  address_offset=hex2dec('00')  intf_name=''  intf_description=''  default_value=0  timing_constraint=None  locs_specified=off  LOCs={}  io_standard={}  inherit_from_input=off  hdl_port=on  dbl_ovrd=off  block_type=gatewayin
  dspsigops_Triggered_Signal_From_Workspace_ch0_data_c{0..3} (4 alike) : xbsIndex_r4/Gateway In  gui_display_data_type=Fixed-point  arith_type=Unsigned  n_bits=10  bin_pt=0  preci_type=Single  exp_width=8  frac_width=24  rows=1  columns=1  quantization=Truncate  overflow=Wrap  period=1  UseAsADC=off  ADCChannel='1'  interface=None  automatic_assignment=on  address_offset=hex2dec('00')  intf_name=''  intf_description=''  default_value=0  timing_constraint=None  locs_specified=off  LOCs={}  io_standard={}  inherit_from_input=off  hdl_port=on  dbl_ovrd=off  block_type=gatewayin
  dspsigops_Triggered_Signal_From_Workspace_ch0_data_d{0..3} (4 alike) : xbsIndex_r4/Gateway In  gui_display_data_type=Fixed-point  arith_type=Unsigned  n_bits=10  bin_pt=0  preci_type=Single  exp_width=8  frac_width=24  rows=1  columns=1  quantization=Truncate  overflow=Wrap  period=1  UseAsADC=off  ADCChannel='1'  interface=None  automatic_assignment=on  address_offset=hex2dec('00')  intf_name=''  intf_description=''  default_value=0  timing_constraint=None  locs_specified=off  LOCs={}  io_standard={}  inherit_from_input=off  hdl_port=on  dbl_ovrd=off  block_type=gatewayin
  dspsigops_Triggered_Signal_From_Workspace_ch1_data_a{0..3} (4 alike) : xbsIndex_r4/Gateway In  gui_display_data_type=Fixed-point  arith_type=Unsigned  n_bits=10  bin_pt=0  preci_type=Single  exp_width=8  frac_width=24  rows=1  columns=1  quantization=Truncate  overflow=Wrap  period=1  UseAsADC=off  ADCChannel='1'  interface=None  automatic_assignment=on  address_offset=hex2dec('00')  intf_name=''  intf_description=''  default_value=0  timing_constraint=None  locs_specified=off  LOCs={}  io_standard={}  inherit_from_input=off  hdl_port=on  dbl_ovrd=off  block_type=gatewayin
  dspsigops_Triggered_Signal_From_Workspace_ch1_data_b{0..3} (4 alike) : xbsIndex_r4/Gateway In  gui_display_data_type=Fixed-point  arith_type=Unsigned  n_bits=10  bin_pt=0  preci_type=Single  exp_width=8  frac_width=24  rows=1  columns=1  quantization=Truncate  overflow=Wrap  period=1  UseAsADC=off  ADCChannel='1'  interface=None  automatic_assignment=on  address_offset=hex2dec('00')  intf_name=''  intf_description=''  default_value=0  timing_constraint=None  locs_specified=off  LOCs={}  io_standard={}  inherit_from_input=off  hdl_port=on  dbl_ovrd=off  block_type=gatewayin
  dspsigops_Triggered_Signal_From_Workspace_ch1_data_c{0..3} (4 alike) : xbsIndex_r4/Gateway In  gui_display_data_type=Fixed-point  arith_type=Unsigned  n_bits=10  bin_pt=0  preci_type=Single  exp_width=8  frac_width=24  rows=1  columns=1  quantization=Truncate  overflow=Wrap  period=1  UseAsADC=off  ADCChannel='1'  interface=None  automatic_assignment=on  address_offset=hex2dec('00')  intf_name=''  intf_description=''  default_value=0  timing_constraint=None  locs_specified=off  LOCs={}  io_standard={}  inherit_from_input=off  hdl_port=on  dbl_ovrd=off  block_type=gatewayin
  dspsigops_Triggered_Signal_From_Workspace_ch1_data_d{0..3} (4 alike) : xbsIndex_r4/Gateway In  gui_display_data_type=Fixed-point  arith_type=Unsigned  n_bits=10  bin_pt=0  preci_type=Single  exp_width=8  frac_width=24  rows=1  columns=1  quantization=Truncate  overflow=Wrap  period=1  UseAsADC=off  ADCChannel='1'  interface=None  automatic_assignment=on  address_offset=hex2dec('00')  intf_name=''  intf_description=''  default_value=0  timing_constraint=None  locs_specified=off  LOCs={}  io_standard={}  inherit_from_input=off  hdl_port=on  dbl_ovrd=off  block_type=gatewayin
  dspsigops_Triggered_Signal_From_Workspace_sync : xbsIndex_r4/Gateway In  gui_display_data_type=Fixed-point  arith_type=Boolean  n_bits=16  bin_pt=14  preci_type=Single  exp_width=8  frac_width=24  rows=1  columns=1  quantization="Round  (unbiased: +/- Inf)"  overflow=Saturate  period=1  UseAsADC=off  ADCChannel='1'  interface=None  automatic_assignment=on  address_offset=hex2dec('00')  intf_name=''  intf_description=''  default_value=0  timing_constraint=None  locs_specified=off  LOCs={}  io_standard={}  inherit_from_input=off  hdl_port=on  dbl_ovrd=off  block_type=gatewayin
  ch0_a0 : Outport
  ch0_a1 : Outport  Port=2
  ch0_a2 : Outport  Port=3
  ch0_a3 : Outport  Port=4
  ch0_b0 : Outport  Port=5
  ch0_b1 : Outport  Port=6
  ch0_b2 : Outport  Port=7
  ch0_b3 : Outport  Port=8
  ch0_c0 : Outport  Port=9
  ch0_c1 : Outport  Port=10
  ch0_c2 : Outport  Port=11
  ch0_c3 : Outport  Port=12
  ch0_d0 : Outport  Port=13
  ch0_d1 : Outport  Port=14
  ch0_d2 : Outport  Port=15
  ch0_d3 : Outport  Port=16
  ch1_a0 : Outport  Port=17
  ch1_a1 : Outport  Port=18
  ch1_a2 : Outport  Port=19
  ch1_a3 : Outport  Port=20
  ch1_b0 : Outport  Port=21
  ch1_b1 : Outport  Port=22
  ch1_b2 : Outport  Port=23
  ch1_b3 : Outport  Port=24
  ch1_c0 : Outport  Port=25
  ch1_c1 : Outport  Port=26
  ch1_c2 : Outport  Port=27
  ch1_c3 : Outport  Port=28
  ch1_d0 : Outport  Port=29
  ch1_d1 : Outport  Port=30
  ch1_d2 : Outport  Port=31
  ch1_d3 : Outport  Port=32
  sync_out : Outport  Port=33
  ad_clk_out : Outport  Port=34
  wires:
  ch0_sim_a/1 -> ch0_gain_a/1
  ch0_gain_a/1 -> ch0_bias_a/1
  ch0_bias_a/1 -> ch0_downsample_a0/1, ch0_downsample_a1/1, ch0_downsample_a2/1, ch0_downsample_a3/1
  ch0_downsample_a0/1 -> ch0_delay_a0/1
  ch0_delay_a0/1 -> dspsigops_Triggered_Signal_From_Workspace_ch0_data_a0/1
  dspsigops_Triggered_Signal_From_Workspace_ch0_data_a0/1 -> ch0_a0/1
  ch0_downsample_a1/1 -> ch0_delay_a1/1
  ch0_delay_a1/1 -> dspsigops_Triggered_Signal_From_Workspace_ch0_data_a1/1
  dspsigops_Triggered_Signal_From_Workspace_ch0_data_a1/1 -> ch0_a1/1
  ch0_downsample_a2/1 -> ch0_delay_a2/1
  ch0_delay_a2/1 -> dspsigops_Triggered_Signal_From_Workspace_ch0_data_a2/1
  dspsigops_Triggered_Signal_From_Workspace_ch0_data_a2/1 -> ch0_a2/1
  ch0_downsample_a3/1 -> ch0_delay_a3/1
  ch0_delay_a3/1 -> dspsigops_Triggered_Signal_From_Workspace_ch0_data_a3/1
  dspsigops_Triggered_Signal_From_Workspace_ch0_data_a3/1 -> ch0_a3/1
  ch0_sim_b/1 -> ch0_gain_b/1
  ch0_gain_b/1 -> ch0_bias_b/1
  ch0_bias_b/1 -> ch0_downsample_b0/1, ch0_downsample_b1/1, ch0_downsample_b2/1, ch0_downsample_b3/1
  ch0_downsample_b0/1 -> ch0_delay_b0/1
  ch0_delay_b0/1 -> dspsigops_Triggered_Signal_From_Workspace_ch0_data_b0/1
  dspsigops_Triggered_Signal_From_Workspace_ch0_data_b0/1 -> ch0_b0/1
  ch0_downsample_b1/1 -> ch0_delay_b1/1
  ch0_delay_b1/1 -> dspsigops_Triggered_Signal_From_Workspace_ch0_data_b1/1
  dspsigops_Triggered_Signal_From_Workspace_ch0_data_b1/1 -> ch0_b1/1
  ch0_downsample_b2/1 -> ch0_delay_b2/1
  ch0_delay_b2/1 -> dspsigops_Triggered_Signal_From_Workspace_ch0_data_b2/1
  dspsigops_Triggered_Signal_From_Workspace_ch0_data_b2/1 -> ch0_b2/1
  ch0_downsample_b3/1 -> ch0_delay_b3/1
  ch0_delay_b3/1 -> dspsigops_Triggered_Signal_From_Workspace_ch0_data_b3/1
  dspsigops_Triggered_Signal_From_Workspace_ch0_data_b3/1 -> ch0_b3/1
  ch0_sim_c/1 -> ch0_gain_c/1
  ch0_gain_c/1 -> ch0_bias_c/1
  ch0_bias_c/1 -> ch0_downsample_c0/1, ch0_downsample_c1/1, ch0_downsample_c2/1, ch0_downsample_c3/1
  ch0_downsample_c0/1 -> ch0_delay_c0/1
  ch0_delay_c0/1 -> dspsigops_Triggered_Signal_From_Workspace_ch0_data_c0/1
  dspsigops_Triggered_Signal_From_Workspace_ch0_data_c0/1 -> ch0_c0/1
  ch0_downsample_c1/1 -> ch0_delay_c1/1
  ch0_delay_c1/1 -> dspsigops_Triggered_Signal_From_Workspace_ch0_data_c1/1
  dspsigops_Triggered_Signal_From_Workspace_ch0_data_c1/1 -> ch0_c1/1
  ch0_downsample_c2/1 -> ch0_delay_c2/1
  ch0_delay_c2/1 -> dspsigops_Triggered_Signal_From_Workspace_ch0_data_c2/1
  dspsigops_Triggered_Signal_From_Workspace_ch0_data_c2/1 -> ch0_c2/1
  ch0_downsample_c3/1 -> ch0_delay_c3/1
  ch0_delay_c3/1 -> dspsigops_Triggered_Signal_From_Workspace_ch0_data_c3/1
  dspsigops_Triggered_Signal_From_Workspace_ch0_data_c3/1 -> ch0_c3/1
  ch0_sim_d/1 -> ch0_gain_d/1
  ch0_gain_d/1 -> ch0_bias_d/1
  ch0_bias_d/1 -> ch0_downsample_d0/1, ch0_downsample_d1/1, ch0_downsample_d2/1, ch0_downsample_d3/1
  ch0_downsample_d0/1 -> ch0_delay_d0/1
  ch0_delay_d0/1 -> dspsigops_Triggered_Signal_From_Workspace_ch0_data_d0/1
  dspsigops_Triggered_Signal_From_Workspace_ch0_data_d0/1 -> ch0_d0/1
  ch0_downsample_d1/1 -> ch0_delay_d1/1
  ch0_delay_d1/1 -> dspsigops_Triggered_Signal_From_Workspace_ch0_data_d1/1
  dspsigops_Triggered_Signal_From_Workspace_ch0_data_d1/1 -> ch0_d1/1
  ch0_downsample_d2/1 -> ch0_delay_d2/1
  ch0_delay_d2/1 -> dspsigops_Triggered_Signal_From_Workspace_ch0_data_d2/1
  dspsigops_Triggered_Signal_From_Workspace_ch0_data_d2/1 -> ch0_d2/1
  ch0_downsample_d3/1 -> ch0_delay_d3/1
  ch0_delay_d3/1 -> dspsigops_Triggered_Signal_From_Workspace_ch0_data_d3/1
  dspsigops_Triggered_Signal_From_Workspace_ch0_data_d3/1 -> ch0_d3/1
  ch1_sim_a/1 -> ch1_gain_a/1
  ch1_gain_a/1 -> ch1_bias_a/1
  ch1_bias_a/1 -> ch1_downsample_a0/1, ch1_downsample_a1/1, ch1_downsample_a2/1, ch1_downsample_a3/1
  ch1_downsample_a0/1 -> ch1_delay_a0/1
  ch1_delay_a0/1 -> dspsigops_Triggered_Signal_From_Workspace_ch1_data_a0/1
  dspsigops_Triggered_Signal_From_Workspace_ch1_data_a0/1 -> ch1_a0/1
  ch1_downsample_a1/1 -> ch1_delay_a1/1
  ch1_delay_a1/1 -> dspsigops_Triggered_Signal_From_Workspace_ch1_data_a1/1
  dspsigops_Triggered_Signal_From_Workspace_ch1_data_a1/1 -> ch1_a1/1
  ch1_downsample_a2/1 -> ch1_delay_a2/1
  ch1_delay_a2/1 -> dspsigops_Triggered_Signal_From_Workspace_ch1_data_a2/1
  dspsigops_Triggered_Signal_From_Workspace_ch1_data_a2/1 -> ch1_a2/1
  ch1_downsample_a3/1 -> ch1_delay_a3/1
  ch1_delay_a3/1 -> dspsigops_Triggered_Signal_From_Workspace_ch1_data_a3/1
  dspsigops_Triggered_Signal_From_Workspace_ch1_data_a3/1 -> ch1_a3/1
  ch1_sim_b/1 -> ch1_gain_b/1
  ch1_gain_b/1 -> ch1_bias_b/1
  ch1_bias_b/1 -> ch1_downsample_b0/1, ch1_downsample_b1/1, ch1_downsample_b2/1, ch1_downsample_b3/1
  ch1_downsample_b0/1 -> ch1_delay_b0/1
  ch1_delay_b0/1 -> dspsigops_Triggered_Signal_From_Workspace_ch1_data_b0/1
  dspsigops_Triggered_Signal_From_Workspace_ch1_data_b0/1 -> ch1_b0/1
  ch1_downsample_b1/1 -> ch1_delay_b1/1
  ch1_delay_b1/1 -> dspsigops_Triggered_Signal_From_Workspace_ch1_data_b1/1
  dspsigops_Triggered_Signal_From_Workspace_ch1_data_b1/1 -> ch1_b1/1
  ch1_downsample_b2/1 -> ch1_delay_b2/1
  ch1_delay_b2/1 -> dspsigops_Triggered_Signal_From_Workspace_ch1_data_b2/1
  dspsigops_Triggered_Signal_From_Workspace_ch1_data_b2/1 -> ch1_b2/1
  ch1_downsample_b3/1 -> ch1_delay_b3/1
  ch1_delay_b3/1 -> dspsigops_Triggered_Signal_From_Workspace_ch1_data_b3/1
  dspsigops_Triggered_Signal_From_Workspace_ch1_data_b3/1 -> ch1_b3/1
  ch1_sim_c/1 -> ch1_gain_c/1
  ch1_gain_c/1 -> ch1_bias_c/1
  ch1_bias_c/1 -> ch1_downsample_c0/1, ch1_downsample_c1/1, ch1_downsample_c2/1, ch1_downsample_c3/1
  ch1_downsample_c0/1 -> ch1_delay_c0/1
  ch1_delay_c0/1 -> dspsigops_Triggered_Signal_From_Workspace_ch1_data_c0/1
  dspsigops_Triggered_Signal_From_Workspace_ch1_data_c0/1 -> ch1_c0/1
  ch1_downsample_c1/1 -> ch1_delay_c1/1
  ch1_delay_c1/1 -> dspsigops_Triggered_Signal_From_Workspace_ch1_data_c1/1
  dspsigops_Triggered_Signal_From_Workspace_ch1_data_c1/1 -> ch1_c1/1
  ch1_downsample_c2/1 -> ch1_delay_c2/1
  ch1_delay_c2/1 -> dspsigops_Triggered_Signal_From_Workspace_ch1_data_c2/1
  dspsigops_Triggered_Signal_From_Workspace_ch1_data_c2/1 -> ch1_c2/1
  ch1_downsample_c3/1 -> ch1_delay_c3/1
  ch1_delay_c3/1 -> dspsigops_Triggered_Signal_From_Workspace_ch1_data_c3/1
  dspsigops_Triggered_Signal_From_Workspace_ch1_data_c3/1 -> ch1_c3/1
  ch1_sim_d/1 -> ch1_gain_d/1
  ch1_gain_d/1 -> ch1_bias_d/1
  ch1_bias_d/1 -> ch1_downsample_d0/1, ch1_downsample_d1/1, ch1_downsample_d2/1, ch1_downsample_d3/1
  ch1_downsample_d0/1 -> ch1_delay_d0/1
  ch1_delay_d0/1 -> dspsigops_Triggered_Signal_From_Workspace_ch1_data_d0/1
  dspsigops_Triggered_Signal_From_Workspace_ch1_data_d0/1 -> ch1_d0/1
  ch1_downsample_d1/1 -> ch1_delay_d1/1
  ch1_delay_d1/1 -> dspsigops_Triggered_Signal_From_Workspace_ch1_data_d1/1
  dspsigops_Triggered_Signal_From_Workspace_ch1_data_d1/1 -> ch1_d1/1
  ch1_downsample_d2/1 -> ch1_delay_d2/1
  ch1_delay_d2/1 -> dspsigops_Triggered_Signal_From_Workspace_ch1_data_d2/1
  dspsigops_Triggered_Signal_From_Workspace_ch1_data_d2/1 -> ch1_d2/1
  ch1_downsample_d3/1 -> ch1_delay_d3/1
  ch1_delay_d3/1 -> dspsigops_Triggered_Signal_From_Workspace_ch1_data_d3/1
  dspsigops_Triggered_Signal_From_Workspace_ch1_data_d3/1 -> ch1_d3/1
  sim_sync/1 -> dspsigops_Triggered_Signal_From_Workspace_sync/1
  dspsigops_Triggered_Signal_From_Workspace_sync/1 -> sync_out/1
  sim_ad_clk/1 -> dspsigops_Triggered_Signal_From_Workspace_ad_clk/1
  dspsigops_Triggered_Signal_From_Workspace_ad_clk/1 -> ad_clk_out/1

== system xps_library/ADCs/adc_mkid ==
  conv : Subsystem
      mask help:
      | Converts an (12-bit) unsigned number to 2's complement.
      | This block should eventually be able to handle arbitrary
      | width inputs.
  conv1 : Subsystem
      mask help:
      | Converts an (12-bit) unsigned number to 2's complement.
      | This block should eventually be able to handle arbitrary
      | width inputs.
  conv2 : Subsystem
      mask help:
      | Converts an (12-bit) unsigned number to 2's complement.
      | This block should eventually be able to handle arbitrary
      | width inputs.
  conv3 : Subsystem
      mask help:
      | Converts an (12-bit) unsigned number to 2's complement.
      | This block should eventually be able to handle arbitrary
      | width inputs.
  xps_library_ADCs_adc_mkid_user_data_i0 : xbsIndex_r4/Gateway In  gui_display_data_type=Fixed-point  arith_type=Unsigned  n_bits=12  bin_pt=0  preci_type=Single  exp_width=8  frac_width=24  rows=1  columns=1  quantization=Truncate  overflow=Wrap  period=1  UseAsADC=off  ADCChannel='1'  interface=None  automatic_assignment=on  address_offset=hex2dec('00')  intf_name=''  intf_description=''  default_value=0  timing_constraint=None  locs_specified=off  LOCs={}  io_standard={}  inherit_from_input=off  hdl_port=on  dbl_ovrd=off  block_type=gatewayin
      settings: infoedit="Gateway in block.  Converts inputs of type Simulink integer, double and fixed point to  Xilinx fixed point type.<P><P>Hardware notes:  In hardware these blocks become top level input ports."  xl_area=[0, 0, 0, 0, 0, 0, 0]  block_version=10.1.3
  xps_library_ADCs_adc_mkid_user_data_i1 : xbsIndex_r4/Gateway In  gui_display_data_type=Fixed-point  arith_type=Unsigned  n_bits=12  bin_pt=0  preci_type=Single  exp_width=8  frac_width=24  rows=1  columns=1  quantization=Truncate  overflow=Wrap  period=1  UseAsADC=off  ADCChannel='1'  interface=None  automatic_assignment=on  address_offset=hex2dec('00')  intf_name=''  intf_description=''  default_value=0  timing_constraint=None  locs_specified=off  LOCs={}  io_standard={}  inherit_from_input=off  hdl_port=on  dbl_ovrd=off  block_type=gatewayin
      settings: infoedit="Gateway in block.  Converts inputs of type Simulink integer, double and fixed point to  Xilinx fixed point type.<P><P>Hardware notes:  In hardware these blocks become top level input ports."  xl_area=[0, 0, 0, 0, 0, 0, 0]  block_version=10.1.3
  xps_library_ADCs_adc_mkid_user_data_q0 : xbsIndex_r4/Gateway In  gui_display_data_type=Fixed-point  arith_type=Unsigned  n_bits=12  bin_pt=0  preci_type=Single  exp_width=8  frac_width=24  rows=1  columns=1  quantization=Truncate  overflow=Wrap  period=1  UseAsADC=off  ADCChannel='1'  interface=None  automatic_assignment=on  address_offset=hex2dec('00')  intf_name=''  intf_description=''  default_value=0  timing_constraint=None  locs_specified=off  LOCs={}  io_standard={}  inherit_from_input=off  hdl_port=on  dbl_ovrd=off  block_type=gatewayin
      settings: infoedit="Gateway in block.  Converts inputs of type Simulink integer, double and fixed point to  Xilinx fixed point type.<P><P>Hardware notes:  In hardware these blocks become top level input ports."  xl_area=[0, 0, 0, 0, 0, 0, 0]  block_version=10.1.3
  xps_library_ADCs_adc_mkid_user_data_q1 : xbsIndex_r4/Gateway In  gui_display_data_type=Fixed-point  arith_type=Unsigned  n_bits=12  bin_pt=0  preci_type=Single  exp_width=8  frac_width=24  rows=1  columns=1  quantization=Truncate  overflow=Wrap  period=1  UseAsADC=off  ADCChannel='1'  interface=None  automatic_assignment=on  address_offset=hex2dec('00')  intf_name=''  intf_description=''  default_value=0  timing_constraint=None  locs_specified=off  LOCs={}  io_standard={}  inherit_from_input=off  hdl_port=on  dbl_ovrd=off  block_type=gatewayin
      settings: infoedit="Gateway in block.  Converts inputs of type Simulink integer, double and fixed point to  Xilinx fixed point type.<P><P>Hardware notes:  In hardware these blocks become top level input ports."  xl_area=[0, 0, 0, 0, 0, 0, 0]  block_version=10.1.3
  xps_library_ADCs_adc_mkid_user_sync : xbsIndex_r4/Gateway In  gui_display_data_type=Fixed-point  arith_type=Boolean  n_bits=1  bin_pt=0  preci_type=Single  exp_width=8  frac_width=24  rows=1  columns=1  quantization=Truncate  overflow=Wrap  period=1  UseAsADC=off  ADCChannel='1'  interface=None  automatic_assignment=on  address_offset=hex2dec('00')  intf_name=''  intf_description=''  default_value=0  timing_constraint=None  locs_specified=off  LOCs={}  io_standard={}  inherit_from_input=off  hdl_port=on  dbl_ovrd=off  block_type=gatewayin
      settings: infoedit="Gateway in block.  Converts inputs of type Simulink integer, double and fixed point to  Xilinx fixed point type.<P><P>Hardware notes:  In hardware these blocks become top level input ports."  xl_area=[0, 0, 0, 0, 0, 0, 0]  block_version=10.1.3
  data_i0 : Outport
  data_i1 : Outport  Port=2
  data_q0 : Outport  Port=3
  data_q1 : Outport  Port=4
  sync : Outport  Port=5
  wires:
  xps_library_ADCs_adc_mkid_user_sync/1 -> sync/1
  xps_library_ADCs_adc_mkid_user_data_i0/1 -> conv/1(In1)
  conv/1(Out1) -> data_i0/1
  xps_library_ADCs_adc_mkid_user_data_q0/1 -> conv2/1(In1)
  conv2/1(Out1) -> data_q0/1
  xps_library_ADCs_adc_mkid_user_data_i1/1 -> conv1/1(In1)
  conv1/1(Out1) -> data_i1/1
  xps_library_ADCs_adc_mkid_user_data_q1/1 -> conv3/1(In1)
  conv3/1(Out1) -> data_q1/1
